simulink model "BDA_DynamicModel_v3"  (R2021b)
settings: Solver=ode23t  StartTime=0.0  StopTime=15  FixedStep=0.000001  MaxStep=1e-5  MinStep=1e-7  RelTol=1e-3
undefined symbols (not defined in the file or in its folder): X, Y, Z
libraries: sm_lib x47, nesl_utility x7
(part 2 of 5)

== matlab function BDA_DynamicModel_v3/Planta/Dinámica Directa/H ==
  data: q2 input; H output; q3 input; q4 input; q5 input; q6 input
function H = H(q2,q3,q4,q5,q6)
%#codegen

%    This function was generated by the Symbolic Math Toolbox version 9.0.
%    28-Nov-2021 14:58:23

t2 = cos(q2);
t3 = cos(q4);
t4 = cos(q5);
t5 = cos(q6);
t6 = sin(q2);
t7 = sin(q4);
t8 = sin(q5);
t9 = sin(q6);
t16 = 9.007199254740992e+15;
t10 = t2.*1.051339e-1;
t11 = t6.*1.051339e-1;
t12 = t4.*5.110348748545983e-1;
t14 = t8.*5.110348748545983e-1;
t15 = t6.*3.235525e-2;
t17 = t2.*3.235525e-2;
t18 = t4.*t7.*8.595599785252598e-1;
t19 = t3.*t9.*8.595599785252598e-1;
t20 = t7.*t8.*8.595599785252598e-1;
t21 = t3.*t5.*8.595599785252598e-1;
t23 = t3.*5.157359871151559e-3;
t24 = t5.*t8.*4.36041e-5;
t25 = t8.*t9.*4.36041e-5;
t26 = (q3.*t16)./9.007199254740992e+15;
t29 = q3.*t16.*1.110223024625157e-16i;
t39 = t5.*1.33637554986e-4;
t40 = t8.*1.33637554986e-4;
t41 = t8.*7.26350557185e-5;
t42 = t9.*7.26350557185e-5;
t43 = t8.*6.1855407534e-5;
t44 = t4.*1.35652563578e-4;
t45 = t3.*t4.*4.990257941055339e-2;
t46 = t5.*t7.*4.990257941055339e-2;
t47 = t7.*t9.*4.990257941055339e-2;
t50 = t4.*t5.*7.26350557185e-5;
t52 = t3.*3.748033925961328e-5;
t53 = t4.*t9.*1.33637554986e-4;
t54 = t3.*t5.*t8.*4.990257941055339e-2;
t55 = t3.*t8.*t9.*4.990257941055339e-2;
t56 = t8.*t9.*4.35810334311e-7;
t61 = t5.*t8.*8.01825329916e-7;
t71 = t6.*5.850606868813307e-5;
t72 = t2.*1.908064240151374e-5;
t74 = t8.*3.161027044821787e-5;
t75 = t8.*3.711904660916042e-5;
t76 = t4.*6.932319085178867e-5;
t77 = t3.*9.395517395143932e-4;
t78 = t7.*9.395517395143932e-4;
t79 = t4.*3.601891949238275e-7;
t80 = t8.*3.601891949238275e-7;
t81 = t3.*5.316843277159623e-5;
t82 = t7.*1.451749445763287e-4;
t83 = t3.*3.746051216014494e-7;
t84 = t3.*1.166015146360021e-4;
t86 = t8.*6.829345118814501e-5;
t89 = t8.*4.203395243364607e-6;
t90 = t7.*5.427853659906482e-4;
t91 = t4.*7.314371377091851e-7;
t92 = t8.*7.314371377091851e-7;
t93 = t3.*t5.*1.148694938939344e-4;
t94 = t5.*3.387428925624357e-6;
t95 = t4.*t7.*6.243418693357491e-5;
t96 = t3.*t9.*6.243418693357491e-5;
t97 = t4.*t7.*1.148694938939344e-4;
t98 = t4.*t7.*5.316843277159623e-5;
t99 = t5.*1.245668607194124e-6;
t100 = t9.*1.745966317740249e-6;
t101 = t9.*1.245668607194124e-6;
t102 = t7.*t8.*1.166015146360021e-4;
t104 = t3.*t4.*5.427853659906482e-4;
t105 = t3.*t8.*5.427853659906482e-4;
t106 = t4.*t7.*6.058377458913066e-7;
t107 = t7.*t8.*6.058377458913066e-7;
t108 = t3.*1.607033050476913e-7;
t109 = t3.*t4.*3.626595104792852e-4;
t110 = t4.*4.0082304082032e-9;
t111 = t5.*t7.*3.626595104792852e-4;
t112 = t7.*t9.*3.626595104792852e-4;
t113 = t4.*t5.*1.745966317740249e-6;
t116 = t3.*6.892169633636063e-7;
t118 = t4.*t9.*3.387428925624357e-6;
t119 = t4.*t9.*(-1.245668607194124e-6);
t120 = t3.*t5.*t8.*3.626595104792852e-4;
t121 = t3.*t8.*t9.*3.626595104792852e-4;
t124 = t8.*5.918087154269792e-7;
t125 = t4.*2.261852897508832e-6;
t132 = t8.*1.87902861198544e-8;
t152 = t4.*3.73789886133219e-7;
t153 = t8.*3.73789886133219e-7;
t154 = t8.*2.148081562157245e-6;
t156 = t7.*6.769412826196288e-6;
t157 = t3.*2.706536467726674e-6;
t158 = t4.*2.048345525044518e-9;
t159 = t3.*2.289498402241797e-6;
t160 = t7.*3.086744386437578e-6;
t162 = t3.*t8.*6.769412826196288e-6;
t163 = t4.*t7.*3.61307032511966e-6;
t165 = t3.*3.445314443599436e-9;
t166 = t4.*t7.*6.287140903818846e-7;
t167 = t7.*t8.*6.287140903818846e-7;
t169 = t3.*t4.*3.086744386437578e-6;
t170 = t3.*t9.*1.500762770582635e-6;
t171 = t3.*t5.*1.070726881249372e-6;
t172 = t3.*t4.*6.668858699921061e-6;
t173 = t3.*t4.*3.624676635982417e-6;
t174 = t3.*t9.*1.070726881249372e-6;
t175 = t5.*t7.*6.668858699921061e-6;
t176 = t7.*6.078899754658124e-9;
t177 = t7.*t9.*3.624676635982417e-6;
t178 = t3.*t5.*2.911698334565516e-6;
t179 = t7.*3.10211731732776e-5;
t180 = t3.*9.392818914088469e-10;
t181 = t7.*9.392818914088469e-10;
t182 = t3.*t4.*3.517249171619401e-8;
t183 = t7.*t8.*3.445314443599436e-9;
t184 = t3.*t8.*3.517249171619401e-8;
t185 = t3.*t5.*t8.*3.624676635982417e-6;
t186 = t3.*t8.*t9.*6.668858699921061e-6;
t190 = t8.*3.024348928260869e-7;
t191 = t4.*1.155885712417937e-6;
t193 = t7.*t8.*1.944198228009988e-6;
t195 = t4.*t7.*5.086950867234759e-7;
t196 = t8.*9.602491515741889e-9;
t207 = t3.*1.615137793366553e-8;
t213 = t4.*t7.*1.615137793366553e-8;
t214 = t3.*2.84449372366336e-5;
t13 = -t11;
t22 = -t20;
t27 = cos(t26);
t28 = sin(t26);
t30 = exp(t29);
t32 = -t29;
t48 = t10+t15;
t49 = -t43;
t57 = -t53;
t58 = -t54;
t59 = t14+t18;
t85 = -t76;
t87 = -t79;
t88 = -t80;
t103 = -t92;
t114 = t4.*t99;
t115 = t4.*t101;
t117 = -t106;
t122 = -t118;
t123 = -t120;
t126 = -t124;
t127 = t23+t45;
t128 = t25+t41;
t129 = t24+t40;
t155 = -t152;
t161 = -t157;
t164 = -t158;
t168 = -t162;
t187 = -t183;
t188 = -t184;
t189 = -t185;
t192 = -t191;
t201 = -t196;
t211 = -t207;
t215 = -t213;
t251 = t39+t42+4.36041e-5;
t266 = t77-8.631097478604537e-5;
t267 = t78+9.554306323645785e-8;
t270 = t82+t108;
t300 = t113+t119;
t314 = t110+t132;
t368 = t56+t61+t89;
t382 = t99+t100+4.35810334311e-7;
t397 = t94+t101+8.01825329916e-7;
t455 = t179+t180+2.208156882018249e-9;
t459 = t181+t214-3.390351827752591e-7;
t31 = t28.^2;
t33 = 1.0./t30;
t34 = t3.*t27;
t35 = t7.*t27;
t36 = t30-1.0;
t51 = t13+t17;
t60 = t12+t22;
t65 = t5.*t59.*(3.0./5.0e+2);
t66 = t9.*t59.*(3.0./5.0e+2);
t67 = t27.*1.273194e-2;
t130 = t5.*t59.*4.36041e-5;
t131 = t9.*t59.*4.36041e-5;
t135 = t27.*3.42298471896e-5;
t136 = t27.*3.07913148585e-5;
t137 = t30.*3.694216783411725e-1;
t138 = t30.*1.305783216588275e-1;
t140 = t27.*3.679077402936e-4;
t194 = t44+t49;
t197 = t3.*t16.*t28.*5.673626844500105e-17;
t198 = t7.*t16.*t28.*5.673626844500105e-17;
t199 = t4.*t16.*t28.*9.543032792050485e-17;
t200 = t8.*t16.*t28.*9.543032792050485e-17;
t203 = t9.*t59.*4.35810334311e-7;
t208 = t50+t57;
t210 = t3.*t16.*t28.*3.404176106700063e-19;
t212 = t5.*t59.*8.01825329916e-7;
t216 = t30.*3.215186923359161e-3;
t218 = t30.*1.345257168956303e-2;
t219 = t27.*8.550795305149304e-7;
t221 = t27.*2.150354518622839e-6;
t228 = t27.*2.380363079699592e-9;
t237 = t16.*t28.*4.87211480085e-18;
t240 = t3.*t16.*t28.*2.479366200131245e-18;
t241 = t7.*t16.*t28.*2.479366200131245e-18;
t242 = t3.*t16.*t28.*7.351481000981246e-18;
t243 = t7.*t16.*t28.*9.810473427588925e-18;
t244 = t7.*t16.*t28.*7.351481000981246e-18;
t245 = t7.*t16.*t28.*4.938358626738924e-18;
t257 = t3.*t16.*t28.*2.47393392290267e-21;
t258 = t30.*1.073174736839591e-5;
t259 = t30.*4.490239736257417e-5;
t262 = t30.*3.887314306731568e-4;
t268 = t16.*t28.*2.127584079327986e-20;
t272 = t16.*t28.*1.611765660673211e-20;
t273 = t8.*t16.*t28.*6.931587185740596e-21;
t274 = t3.*t16.*t28.*7.696420262413979e-21;
t277 = t3.*t16.*t28.*3.509445006623964e-21;
t278 = t4.*t16.*t28.*1.294536862550567e-20;
t279 = t7.*t16.*t28.*5.371403294717661e-20;
t280 = t3.*t16.*t28.*2.472625211857455e-23;
t283 = t8.*t16.*t28.*1.275307569480848e-20;
t284 = t7.*t16.*t28.*9.582443148530891e-21;
t285 = t8.*t16.*t28.*5.902881824626087e-21;
t288 = t4.*t16.*t28.*6.726150146755334e-23;
t289 = t8.*t16.*t28.*6.726150146755334e-23;
t290 = t16.*t28.*1.78416509397307e-23;
t292 = t3.*t16.*t28.*2.503226128461205e-19;
t293 = t7.*t16.*t28.*2.503226128461205e-19;
t294 = t3.*t16.*t28.*1.095358398302466e-19;
t295 = t7.*t16.*t28.*1.06707538424542e-19;
t296 = t7.*t16.*t28.*1.095358398302466e-19;
t298 = t114+t122;
t303 = t3.*t16.*t28.*4.549257716411571e-23;
t304 = t3.*t16.*t28.*1.060741086483328e-23;
t305 = t91+t126;
t306 = t103+t125;
t308 = t16.*t28.*t48.*5.673626844500105e-17;
t311 = t30.*5.594793061269655e-7;
t315 = t30.*2.27206524062708e-6;
t318 = t30.*2.515092356455324e-9;
t322 = t16.*t28.*2.00574854081142e-22;
t323 = t16.*t28.*2.258468230849856e-22;
t324 = t16.*t28.*6.331121467597849e-23;
t326 = t7.*t16.*t28.*1.330815870366286e-21;
t327 = t7.*t16.*t28.*6.699010075846667e-22;
t328 = t4.*t16.*t28.*6.980128590482299e-23;
t329 = t8.*t16.*t28.*6.980128590482299e-23;
t330 = t8.*t16.*t28.*4.011313864537747e-22;
t332 = t7.*t16.*t28.*3.054641854059808e-22;
t333 = t7.*t16.*t28.*6.068308319649908e-22;
t334 = t4.*t16.*t28.*3.825067422357704e-25;
t335 = t3.*t16.*t28.*1.511210377393976e-22;
t340 = t3.*t16.*t28.*4.563917575948183e-22;
t341 = t3.*t16.*t28.*2.274120364292329e-25;
t342 = t16.*t28.*t48.*1.893760189037778e-19;
t343 = t16.*t28.*4.123498135247176e-25;
t346 = t7.*t16.*t28.*3.145845434116526e-21;
t347 = t3.*t16.*t28.*1.279265104253459e-21;
t350 = t7.*t16.*t28.*6.39965864882112e-21;
t351 = t7.*t16.*t28.*7.086968837016952e-25;
t353 = t3.*t16.*t28.*6.199840717099487e-26;
t354 = t7.*t16.*t28.*6.199840717099487e-26;
t360 = t7.*t16.*t28.*1.6195873051144e-24;
t362 = t4.*t16.*t28.*2.158493637172119e-22;
t363 = t8.*t16.*t28.*5.647649977940937e-23;
t367 = t3.*t16.*t28.*1.659646412768137e-22;
t370 = t3.*t16.*t28.*1.066090717454436e-24;
t371 = t16.*t28.*3.909932369564116e-22;
t372 = t8.*t16.*t28.*1.793163166137816e-24;
t373 = t3.*t16.*t28.*2.975797947808626e-21;
t375 = t3.*t16.*t28.*6.22961116251322e-21;
t380 = t16.*t28.*5.699051429514929e-23;
t385 = t16.*t28.*t48.*1.94207379898051e-21;
t387 = t16.*t28.*t48.*1.746984305586406e-21;
t405 = t16.*t28.*1.428206656218648e-22;
t412 = t16.*t28.*t48.*5.091703513734173e-22;
t456 = t81+t87+t104+t107;
t457 = t84+t88+t105+t117;
t458 = t161+t176+2.093791190610393e-6;
t487 = t74+t85+t90+t98+t102;
t580 = t153+t156+t165+t166+t182+t192+t193;
t581 = t155+t160+t167+t188+t190+t195+t211;
t582 = t159+t162+t164+t169+t183+t201+t215;
t37 = t36.^2;
t38 = t35.*(3.0./5.0e+2);
t62 = t5.*t60;
t63 = t9.*t60;
t68 = t34.*2.228474e-2;
t69 = t35.*2.228474e-2;
t70 = t34.*6.562549e-2;
t73 = t35.*4.36041e-5;
t139 = t33.*3.694216783411725e-1;
t141 = t33.*1.305783216588275e-1;
t142 = t34.*1.3117937708872e-3;
t143 = t35.*1.3117937708872e-3;
t144 = t35.*1.35652563578e-4;
t145 = t34.*1.688944904408e-4;
t146 = t35.*6.1855407534e-5;
t147 = t35.*4.35810334311e-7;
t148 = t34.*7.13801892181e-4;
t149 = t35.*1.869599668e-7;
t151 = t35.*8.01825329916e-7;
t205 = -t198;
t206 = -t199;
t217 = t33.*3.215186923359161e-3;
t220 = t33.*1.345257168956303e-2;
t222 = t34.*8.902265954562403e-6;
t223 = t35.*4.427198467956924e-6;
t225 = t35.*2.663570267859459e-6;
t226 = t34.*4.059291428568442e-6;
t227 = t35.*4.0082304082032e-9;
t230 = t34.*4.114486328260564e-5;
t231 = t34.*8.487305697640184e-9;
t232 = t34.*1.092747353151976e-9;
t233 = t35.*1.092747353151976e-9;
t235 = t35.*2.925194867859459e-6;
t236 = t35.*1.87902861198544e-8;
t238 = t35.*3.814770659661843e-5;
t246 = -t241;
t252 = -t243;
t253 = -t244;
t254 = -t245;
t260 = t33.*1.073174736839591e-5;
t261 = t33.*4.490239736257417e-5;
t263 = t33.*3.887314306731568e-4;
t264 = t35.*2.262452815028836e-6;
t265 = t34.*4.33730920504627e-9;
t269 = t35+t197;
t286 = -t278;
t287 = -t279;
t297 = -t284;
t299 = -t293;
t301 = -t295;
t302 = -t296;
t307 = -t304;
t309 = t16.*t28.*t51.*9.543032792050485e-17;
t312 = t33.*5.594793061269655e-7;
t317 = t33.*2.27206524062708e-6;
t319 = t33.*2.515092356455324e-9;
t320 = t46+t55+t65;
t321 = t47+t58+t66;
t325 = -t324;
t331 = -t326;
t336 = -t328;
t338 = -t329;
t344 = -t332;
t345 = -t333;
t348 = -t341;
t349 = -t346;
t352 = t16.*t28.*t51.*3.185302114428987e-19;
t355 = -t350;
t356 = -t351;
t358 = -t353;
t359 = -t354;
t361 = -t360;
t365 = -t362;
t374 = -t373;
t376 = -t375;
t381 = -t380;
t390 = t16.*t28.*t51.*3.266565541972299e-21;
t398 = t16.*t28.*t51.*2.938425274050169e-21;
t413 = t16.*t28.*t51.*8.564238525144865e-22;
t414 = -t412;
t488 = t75+t95+t112+t123+t131;
t489 = t86+t97+t111+t121+t130;
t490 = t16.*t28.*t458.*9.543032792050485e-17;
t594 = t154+t163+t175+t177+t186+t189+t203+t212;
t64 = -t62;
t133 = t21+t63;
t150 = -t149;
t202 = t63.*1.33637554986e-4;
t204 = t62.*7.26350557185e-5;
t224 = -t222;
t229 = -t227;
t234 = -t233;
t239 = -t238;
t247 = t63.*3.387428925624357e-6;
t248 = t62.*1.745966317740249e-6;
t249 = t62.*1.245668607194124e-6;
t250 = t63.*1.245668607194124e-6;
t271 = t34+t205;
t275 = t5.*t269;
t276 = t9.*t269;
t310 = -t309;
t313 = t33.*t37.*7.997968101822611e-3;
t316 = t33.*t37.*5.407940120688672e-3;
t337 = t4.*t269.*4.334075e-2;
t339 = t8.*t269.*4.334075e-2;
t357 = -t352;
t364 = t33.*t37.*2.669585786930656e-5;
t366 = t33.*t37.*1.805078477303827e-5;
t369 = t33.*t37.*1.56270217221073e-4;
t377 = t33.*t37.*t48.*2.196325630278387e-1;
t378 = t33.*t37.*t51.*2.196325630278387e-1;
t383 = t4.*t269.*4.71413003675e-4;
t384 = t8.*t269.*4.71413003675e-4;
t386 = t39.*t269;
t388 = t4.*t269.*3.149723995125e-4;
t389 = t42.*t269;
t396 = -t390;
t401 = -t398;
t404 = t33.*t37.*4.313809179931398e-7;
t406 = t33.*t37.*9.133712910180717e-7;
t407 = t33.*t37.*1.011068305420342e-9;
t408 = t33.*t37.*t48.*7.330961578512107e-4;
t409 = t33.*t37.*t51.*7.330961578512107e-4;
t410 = t33.*t37.*t48.*6.346599179580158e-3;
t415 = t4.*t269.*3.148057791131579e-6;
t416 = t8.*t269.*5.879283844893203e-6;
t417 = t4.*t269.*2.68085975407921e-6;
t418 = t4.*t269.*5.791951861259479e-6;
t419 = t94.*t269;
t420 = t4.*t269.*4.57069415115421e-6;
t422 = t99.*t269;
t423 = t100.*t269;
t424 = t101.*t269;
t426 = t4.*t269.*3.054756263814e-8;
t428 = t8.*t269.*3.054756263814e-8;
t433 = t137+t139+2.61156643317655e-1;
t434 = t138+t141+7.38843356682345e-1;
t438 = t33.*t37.*t48.*7.517989070303108e-6;
t440 = t33.*t37.*t51.*6.762775401369527e-6;
t442 = t33.*t37.*t48.*3.70947298167937e-5;
t443 = t33.*t37.*t48.*4.106249669188362e-8;
t466 = t269.*t314;
t503 = t269.*t459;
t595 = t269.*t582;
t134 = t19+t64;
t209 = -t204;
t255 = -t248;
t256 = -t249;
t281 = t4.*t271;
t282 = t8.*t271;
t291 = -t276;
t379 = -t378;
t393 = t276.*4.35810334311e-7;
t402 = t275.*8.01825329916e-7;
t411 = -t409;
t425 = t91.*t271;
t427 = t92.*t271;
t430 = -t426;
t441 = -t440;
t450 = t48.*t434;
t451 = t51.*t433;
t497 = t237+t308+t310;
t502 = t271.*t455;
t504 = -t503;
t505 = t216+t217+t313+1.819229615328168e-2;
t506 = t218+t220+t316+9.510076620873934e-3;
t528 = t268+t342+t357;
t555 = t323+t385+t396;
t558 = t322+t387+t401;
t563 = t136+t258+t260+t364+6.072279186930818e-5;
t564 = t135+t259+t261+t366+3.174301904745164e-5;
t592 = t219+t311+t312+t404+8.856931883486768e-7;
t596 = -t595;
t639 = t140+t145+t150+t262+t263+t297+t307+t369+2.748073584704864e-4;
t391 = t282.*1.35652563578e-4;
t392 = t281.*1.33637554986e-4;
t394 = t281.*7.26350557185e-5;
t395 = t281.*6.1855407534e-5;
t399 = t281.*7.0482312e-7;
t400 = t282.*7.0482312e-7;
t421 = t281.*4.203395243364607e-6;
t429 = t281.*(-7.314371377091851e-7);
t431 = t282.*4.0082304082032e-9;
t435 = t281.*5.918087154269792e-7;
t436 = t282.*2.261852897508832e-6;
t439 = t281.*1.87902861198544e-8;
t444 = t200+t281;
t445 = t206+t282;
t446 = -t5.*(t199-t282);
t447 = -t9.*(t199-t282);
t452 = -t451;
t460 = t450.*3.33783e-3;
t461 = t451.*3.33783e-3;
t462 = t451.*2.889644e-2;
t465 = t9.*(t199-t282).*(-1.33637554986e-4);
t468 = t5.*(t199-t282).*(-7.26350557185e-5);
t469 = t5.*(t199-t282).*(-4.35810334311e-7);
t470 = t5.*(t199-t282).*7.26350557185e-5;
t471 = t5.*(t199-t282).*4.35810334311e-7;
t473 = t9.*(t199-t282).*(-8.01825329916e-7);
t474 = t451.*3.42298471896e-5;
t475 = t450.*3.07913148585e-5;
t477 = t451.*1.688944904408e-4;
t479 = t451.*1.869599668e-7;
t481 = t9.*(t199-t282).*(-3.387428925624357e-6);
t482 = t5.*(t199-t282).*(-1.745966317740249e-6);
t483 = -t99.*(t199-t282);
t484 = -t101.*(t199-t282);
t485 = t5.*(t199-t282).*1.745966317740249e-6;
t486 = t5.*(t199-t282).*1.245668607194124e-6;
t493 = -t306.*(t199-t282);
t496 = t306.*(t199-t282);
t498 = t3.*t497;
t499 = t7.*t497;
t507 = t3.*t505;
t508 = t7.*t505;
H = ft_1({t105,t106,t109,t116,t127,t128,t129,t133,t134,t142,t143,t144,t146,t147,t148,t151,t158,t159,t16,t168,t169,t170,t171,t172,t173,t174,t178,t187,t196,t199,t2,t202,t208,t209,t210,t213,t221,t222,t223,t224,t225,t226,t227,t228,t229,t230,t231,t232,t234,t235,t236,t237,t239,t240,t242,t246,t247,t250,t251,t252,t253,t254,t255,t256,t257,t264,t265,t266,t267,t268,t269,t27,t270,t271,t272,t273,t274,t275,t276,t277,t28,t280,t282,t283,t285,t286,t287,t288,t289,t290,t291,t292,t294,t298,t299,t3,t300,t301,t302,t303,t305,t306,t31,t314,t315,t317,t318,t319,t320,t321,t325,t326,t327,t329,t330,t331,t334,t335,t336,t337,t338,t339,t340,t341,t343,t344,t345,t347,t348,t349,t355,t356,t358,t359,t361,t362,t363,t365,t367,t368,t370,t371,t372,t374,t376,t377,t379,t38,t381,t382,t383,t384,t386,t388,t389,t39,t391,t392,t393,t394,t395,t397,t399,t4,t40,t400,t402,t405,t406,t407,t408,t41,t410,t411,t413,t414,t415,t416,t417,t418,t419,t42,t420,t421,t422,t423,t424,t425,t426,t427,t428,t429,t43,t430,t431,t435,t436,t438,t439,t44,t441,t442,t443,t444,t446,t447,t45,t450,t452,t455,t456,t458,t459,t460,t461,t462,t465,t466,t470,t471,t473,t474,t475,t477,t479,t48,t481,t484,t485,t486,t487,t488,t489,t490,t496,t497,t498,t499,t5,t502,t504,t505,t506,t507,t508,t51,t52,t528,t555,t558,t563,t564,t580,t581,t582,t59,t592,t594,t596,t6,t60,t62,t63,t639,t67,t68,t69,t7,t70,t71,t72,t73,t8,t80,t83,t84,t9,t93,t96});
end
function H = ft_1(ct)
t105 = ct{1};
t106 = ct{2};
t109 = ct{3};
t116 = ct{4};
t127 = ct{5};
t128 = ct{6};
t129 = ct{7};
t133 = ct{8};
t134 = ct{9};
t142 = ct{10};
t143 = ct{11};
t144 = ct{12};
t146 = ct{13};
t147 = ct{14};
t148 = ct{15};
t151 = ct{16};
t158 = ct{17};
t159 = ct{18};
t16 = ct{19};
t168 = ct{20};
t169 = ct{21};
t170 = ct{22};
t171 = ct{23};
t172 = ct{24};
t173 = ct{25};
t174 = ct{26};
t178 = ct{27};
t187 = ct{28};
t196 = ct{29};
t199 = ct{30};
t2 = ct{31};
t202 = ct{32};
t208 = ct{33};
t209 = ct{34};
t210 = ct{35};
t213 = ct{36};
t221 = ct{37};
t222 = ct{38};
t223 = ct{39};
t224 = ct{40};
t225 = ct{41};
t226 = ct{42};
t227 = ct{43};
t228 = ct{44};
t229 = ct{45};
t230 = ct{46};
t231 = ct{47};
t232 = ct{48};
t234 = ct{49};
t235 = ct{50};
t236 = ct{51};
t237 = ct{52};
t239 = ct{53};
t240 = ct{54};
t242 = ct{55};
t246 = ct{56};
t247 = ct{57};
t250 = ct{58};
t251 = ct{59};
t252 = ct{60};
t253 = ct{61};
t254 = ct{62};
t255 = ct{63};
t256 = ct{64};
t257 = ct{65};
t264 = ct{66};
t265 = ct{67};
t266 = ct{68};
t267 = ct{69};
t268 = ct{70};
t269 = ct{71};
t27 = ct{72};
t270 = ct{73};
t271 = ct{74};
t272 = ct{75};
t273 = ct{76};
t274 = ct{77};
t275 = ct{78};
t276 = ct{79};
t277 = ct{80};
t28 = ct{81};
t280 = ct{82};
t282 = ct{83};
t283 = ct{84};
t285 = ct{85};
t286 = ct{86};
t287 = ct{87};
t288 = ct{88};
t289 = ct{89};
t290 = ct{90};
t291 = ct{91};
t292 = ct{92};
t294 = ct{93};
t298 = ct{94};
t299 = ct{95};
t3 = ct{96};
t300 = ct{97};
t301 = ct{98};
t302 = ct{99};
t303 = ct{100};
t305 = ct{101};
t306 = ct{102};
t31 = ct{103};
t314 = ct{104};
t315 = ct{105};
t317 = ct{106};
t318 = ct{107};
t319 = ct{108};
t320 = ct{109};
t321 = ct{110};
t325 = ct{111};
t326 = ct{112};
t327 = ct{113};
t329 = ct{114};
t330 = ct{115};
t331 = ct{116};
t334 = ct{117};
t335 = ct{118};
t336 = ct{119};
t337 = ct{120};
t338 = ct{121};
t339 = ct{122};
t340 = ct{123};
t341 = ct{124};
t343 = ct{125};
t344 = ct{126};
t345 = ct{127};
t347 = ct{128};
t348 = ct{129};
t349 = ct{130};
t355 = ct{131};
t356 = ct{132};
t358 = ct{133};
t359 = ct{134};
t361 = ct{135};
t362 = ct{136};
t363 = ct{137};
t365 = ct{138};
t367 = ct{139};
t368 = ct{140};
t370 = ct{141};
t371 = ct{142};
t372 = ct{143};
t374 = ct{144};
t376 = ct{145};
t377 = ct{146};
t379 = ct{147};
t38 = ct{148};
t381 = ct{149};
t382 = ct{150};
t383 = ct{151};
t384 = ct{152};
t386 = ct{153};
t388 = ct{154};
t389 = ct{155};
t39 = ct{156};
t391 = ct{157};
t392 = ct{158};
t393 = ct{159};
t394 = ct{160};
t395 = ct{161};
t397 = ct{162};
t399 = ct{163};
t4 = ct{164};
t40 = ct{165};
t400 = ct{166};
t402 = ct{167};
t405 = ct{168};
t406 = ct{169};
t407 = ct{170};
t408 = ct{171};
t41 = ct{172};
t410 = ct{173};
t411 = ct{174};
t413 = ct{175};
t414 = ct{176};
t415 = ct{177};
t416 = ct{178};
t417 = ct{179};
t418 = ct{180};
t419 = ct{181};
t42 = ct{182};
t420 = ct{183};
t421 = ct{184};
t422 = ct{185};
t423 = ct{186};
t424 = ct{187};
t425 = ct{188};
t426 = ct{189};
t427 = ct{190};
t428 = ct{191};
t429 = ct{192};
t43 = ct{193};
t430 = ct{194};
t431 = ct{195};
t435 = ct{196};
t436 = ct{197};
t438 = ct{198};
t439 = ct{199};
t44 = ct{200};
t441 = ct{201};
t442 = ct{202};
t443 = ct{203};
t444 = ct{204};
t446 = ct{205};
t447 = ct{206};
t45 = ct{207};
t450 = ct{208};
t452 = ct{209};
t455 = ct{210};
t456 = ct{211};
t458 = ct{212};
t459 = ct{213};
t460 = ct{214};
t461 = ct{215};
t462 = ct{216};
t465 = ct{217};
t466 = ct{218};
t470 = ct{219};
t471 = ct{220};
t473 = ct{221};
t474 = ct{222};
t475 = ct{223};
t477 = ct{224};
t479 = ct{225};
t48 = ct{226};
t481 = ct{227};
t484 = ct{228};
t485 = ct{229};
t486 = ct{230};
t487 = ct{231};
t488 = ct{232};
t489 = ct{233};
t490 = ct{234};
t496 = ct{235};
t497 = ct{236};
t498 = ct{237};
t499 = ct{238};
t5 = ct{239};
t502 = ct{240};
t504 = ct{241};
t505 = ct{242};
t506 = ct{243};
t507 = ct{244};
t508 = ct{245};
t51 = ct{246};
t52 = ct{247};
t528 = ct{248};
t555 = ct{249};
t558 = ct{250};
t563 = ct{251};
t564 = ct{252};
t580 = ct{253};
t581 = ct{254};
t582 = ct{255};
t59 = ct{256};
t592 = ct{257};
t594 = ct{258};
t596 = ct{259};
t6 = ct{260};
t60 = ct{261};
t62 = ct{262};
t63 = ct{263};
t639 = ct{264};
t67 = ct{265};
t68 = ct{266};
t69 = ct{267};
t7 = ct{268};
t70 = ct{269};
t71 = ct{270};
t72 = ct{271};
t73 = ct{272};
t8 = ct{273};
t80 = ct{274};
t83 = ct{275};
t84 = ct{276};
t9 = ct{277};
t93 = ct{278};
t96 = ct{279};
t525 = t52+t93+t96+t109+t202+t209;
t536 = t67+t506;
t546 = -t300.*(t276+t5.*(t199-t282));
t547 = t300.*(t276+t5.*(t199-t282));
t559 = -t382.*(t276+t5.*(t199-t282));
t561 = t382.*(t276+t5.*(t199-t282));
t562 = t83+t170+t171+t173+t250+t255;
t565 = t116+t172+t174+t178+t247+t256;
t573 = t16.*t28.*t555.*9.543032792050485e-17;
t574 = t16.*t28.*t558.*5.673626844500105e-17;
t593 = t27.*t592;
t599 = t379+t450+t505;
t605 = -t580.*(t199-t282);
t403 = -t400;
t432 = -t431;
t437 = -t436;
t448 = t5.*t444.*(3.0./5.0e+2);
t449 = t9.*t444.*(3.0./5.0e+2);
t453 = t5.*t444.*4.36041e-5;
t454 = t9.*t444.*4.36041e-5;
t463 = -t461;
t464 = -t462;
t467 = t9.*t444.*4.35810334311e-7;
t472 = t5.*t444.*8.01825329916e-7;
t476 = -t474;
t478 = -t477;
t480 = -t479;
t491 = t275+t447;
t492 = t305.*t444;
t494 = t291+t446;
t500 = -t499;
t501 = t368.*t444;
t509 = t498.*2.889644e-2;
t510 = t499.*2.889644e-2;
t512 = t499.*1.08769e-2;
t514 = t507.*2.889644e-2;
t515 = t508.*2.889644e-2;
t516 = t507.*1.08769e-2;
t517 = t498.*1.688944904408e-4;
t518 = t499.*6.1855407534e-5;
t519 = t498.*6.678441185616e-4;
t520 = t499.*6.678441185616e-4;
t521 = t499.*1.35652563578e-4;
t526 = t499.*1.869599668e-7;
t529 = t508.*1.688944904408e-4;
t530 = t507.*6.1855407534e-5;
t531 = t507.*6.678441185616e-4;
t532 = t508.*6.678441185616e-4;
t533 = t507.*1.35652563578e-4;
t535 = t507.*1.869599668e-7;
t537 = t8.*t536;
t538 = t4.*t536;
t548 = t41.*t536;
t549 = t43.*t536;
t550 = t44.*t536;
t551 = t40.*t536;
t566 = t69+t242+t508;
t567 = t68+t253+t507;
t568 = t70+t252+t507;
t600 = t377+t452+t506;
t601 = t3.*t599;
t602 = t7.*t599;
t607 = t444.*t581;
t616 = t377+t452+t536;
t625 = -t562.*(t276+t5.*(t199-t282));
t638 = t444.*t594;
t640 = t411+t460+t563;
t495 = -t492;
t511 = -t510;
t513 = -t512;
t522 = -t518;
t523 = -t519;
t524 = -t520;
t527 = -t526;
t534 = -t532;
t539 = -t537;
t540 = t537.*7.26735e-3;
t541 = t538.*1.08769e-2;
t542 = t537.*1.08769e-2;
t545 = t298.*t491;
t552 = t537.*(-7.26350557185e-5);
t553 = t537.*(-6.1855407534e-5);
t554 = t537.*(-1.33637554986e-4);
t556 = t538.*7.0482312e-7;
t557 = t537.*7.0482312e-7;
t560 = t397.*t491;
t569 = t4.*t566;
t570 = t8.*t566;
t571 = t5.*t568;
t572 = t9.*t568;
t587 = t39.*t568;
t588 = t42.*t568;
t597 = t143+t272+t292+t515;
t598 = t142+t290+t299+t514;
t603 = t601.*2.889644e-2;
t604 = t602.*2.889644e-2;
t606 = t601.*1.08769e-2;
t608 = t602.*1.688944904408e-4;
t609 = t601.*6.1855407534e-5;
t610 = t601.*6.678441185616e-4;
t611 = t602.*6.678441185616e-4;
t612 = t601.*1.35652563578e-4;
t615 = t601.*1.869599668e-7;
t617 = t4.*t616;
t618 = t8.*t616;
t626 = t44.*t616;
t627 = t40.*t616;
t628 = t41.*t616;
t629 = t43.*t616;
t633 = t491.*t565;
t641 = t408+t463+t564;
t653 = t148+t285+t286+t301+t391+t395+t516;
t655 = t69+t240+t498+t602;
t658 = t68+t246+t500+t601;
t659 = t70+t254+t500+t601;
t675 = t410+t464+t639;
t676 = t223+t231+t347+t361+t371+t529+t535;
t679 = t438+t441+t475+t476+t592;
t684 = t221+t230+t234+t315+t317+t343+t355+t358+t406+t531+1.606199544935468e-6;
t543 = -t540;
t544 = -t542;
t575 = t570.*1.08769e-2;
t576 = t569.*7.26735e-3;
t577 = t569.*1.08769e-2;
t578 = t571.*7.26735e-3;
t579 = t572.*7.26735e-3;
t583 = t569.*1.33637554986e-4;
t584 = t569.*7.26350557185e-5;
t585 = t569.*6.1855407534e-5;
t586 = t570.*1.35652563578e-4;
t589 = t569.*7.0482312e-7;
t590 = t570.*7.0482312e-7;
t613 = -t611;
t614 = -t612;
t619 = -t618;
t620 = t617.*1.08769e-2;
t621 = t618.*1.08769e-2;
t622 = t618.*7.26735e-3;
t630 = t618.*(-1.33637554986e-4);
t631 = t618.*(-7.26350557185e-5);
t632 = t618.*(-6.1855407534e-5);
t634 = t618.*7.0482312e-7;
t635 = t617.*7.0482312e-7;
t637 = -t633;
t642 = t339+t538+t570;
t643 = t337+t539+t569;
t656 = t4.*t655;
t657 = t8.*t655;
t660 = t5.*t659;
t661 = t9.*t659;
t673 = t39.*t659;
t674 = t42.*t659;
t677 = t143+t272+t294+t509+t604;
t678 = t142+t290+t302+t511+t603;
t680 = t16.*t28.*t676.*9.543032792050485e-17;
t681 = t27.*t679;
t685 = t228+t232+t239+t318+t319+t325+t359+t376+t407+t534+1.778003609304047e-9;
t686 = t271.*t684;
t691 = t148+t285+t286+t287+t391+t395+t513+t606;
t716 = t221+t230+t234+t315+t317+t343+t349+t358+t406+t442+t478+t524+t610+1.606199544935468e-6;
t720 = t223+t231+t340+t356+t371+t517+t527+t608+t615;
t591 = -t589;
t623 = -t621;
t624 = -t622;
t636 = -t634;
t644 = t5.*t642;
t645 = t9.*t642;
t654 = t38+t210+t643;
t662 = t656.*7.26735e-3;
t663 = t656.*1.08769e-2;
t664 = t657.*1.08769e-2;
t665 = t660.*7.26735e-3;
t666 = t661.*7.26735e-3;
t667 = t656.*7.26350557185e-5;
t668 = t656.*6.1855407534e-5;
t669 = t657.*1.35652563578e-4;
t670 = t656.*1.33637554986e-4;
t671 = t656.*7.0482312e-7;
t672 = t657.*7.0482312e-7;
t682 = t144+t274+t289+t384+t399+t541+t575;
t683 = t146+t277+t288+t383+t403+t544+t577;
t687 = t269.*t685;
t692 = t73+t257+t386+t388+t389+t465+t470+t543+t576;
t695 = t339+t617+t657;
t696 = t337+t619+t656;
t706 = t147+t280+t415+t422+t423+t484+t485+t552+t584;
t707 = t151+t303+t418+t419+t424+t481+t486+t554+t583;
t715 = t226+t236+t336+t345+t363+t370+t427+t428+t435+t530+t556+t590;
t717 = t228+t232+t239+t318+t319+t325+t359+t374+t407+t443+t480+t523+t613+1.778003609304047e-9;
t718 = (t199-t282).*(t224+t227+t326+t338+t341+t362-t425+t426+t437-t533-t557+t589);
t721 = t271.*t716;
t724 = t16.*t28.*t720.*9.543032792050485e-17;
t726 = t225+t334+t335+t372+t416+t417+t432+t439+t550+t553+t585+t586;
t646 = -t645;
t647 = t644.*7.26735e-3;
t648 = t645.*7.26735e-3;
t650 = t645.*1.33637554986e-4;
t651 = t644.*7.26350557185e-5;
t688 = -t687;
t689 = t449+t572+t644;
t697 = t5.*t695;
t698 = t9.*t695;
t708 = t38+t210+t696;
t709 = -t706.*(t276+t5.*(t199-t282));
t710 = t706.*(t276+t5.*(t199-t282));
t711 = t491.*t707;
t712 = t222+t229+t329+t331+t348+t365+t425+t430+t436+t533+t557+t591;
t713 = t144+t274+t289+t384+t399+t620+t664;
t714 = t146+t277+t288+t383+t403+t623+t663;
t719 = t444.*t715;
t722 = t269.*t717;
t725 = t73+t257+t386+t388+t389+t465+t470+t624+t662;
t727 = t147+t280+t415+t422+t423+t484+t485+t631+t667;
t728 = t151+t303+t418+t419+t424+t481+t486+t630+t670;
t729 = t269.*t726;
t739 = t224+t227+t327+t338+t341+t362+t426+t429+t437+t521+t614+t636+t671;
t740 = t226+t236+t336+t344+t363+t370+t427+t428+t435+t522+t609+t635+t672;
t744 = t225+t334+t335+t372+t416+t417+t432+t439+t626+t632+t668+t669;
t649 = -t648;
t652 = -t650;
t690 = t448+t571+t646;
t693 = t273+t394+t454+t579+t647;
t699 = -t698;
t700 = t697.*7.26735e-3;
t701 = t698.*7.26735e-3;
t703 = t698.*1.33637554986e-4;
t704 = t697.*7.26350557185e-5;
t723 = -t722;
t730 = t449+t661+t697;
t732 = -t727.*(t276+t5.*(t199-t282));
t733 = t727.*(t276+t5.*(t199-t282));
t734 = t491.*t728;
t741 = -t739.*(t199-t282);
t742 = t739.*(t199-t282);
t743 = t444.*t740;
t745 = t269.*t744;
t694 = t283+t392+t453+t578+t649;
t702 = -t701;
t705 = -t703;
t731 = t448+t660+t699;
t735 = t273+t394+t454+t666+t700;
t737 = t330+t421+t467+t472+t587+t588+t651+t652;
t736 = t283+t392+t453+t665+t702;
t738 = t444.*t737;
t746 = t330+t421+t467+t472+t673+t674+t704+t705;
t747 = t444.*t746;
et1 = t2.*(-6.595899203175001e-4)+t6.*2.143246017993e-3;
et2 = 4.573233567645e-4;
et3 = t71+t72+t573+t574+t681+t721+t723+t724+t733+t734+t742+t743+t745+t747+t497.*t528+t599.*t640+t600.*t641+t616.*t675+t655.*t677+t658.*t678+t659.*t691+t695.*t713+t696.*t714+t708.*t725+t730.*t735+t731.*t736-t51.*(et1+et2);
et4 = t48.*(t2.*2.143246017993e-3+t6.*6.595899203175001e-4+3.222314966007e-4);
et5 = 2.531318772537663e-4;
et6 = t264+t265+t405+t413+t414+t498.*8.631097478604537e-5;
et7 = t499.*(-9.554306323645785e-8);
et8 = t601.*9.554306323645785e-8;
et9 = t602.*8.631097478604537e-5-t3.*t677.*1.264860527128474e-2;
et10 = t7.*t678.*1.264860527128474e-2+t7.*t691.*4.990257941055339e-2+t3.*t717.*8.595599785252598e-1;
et11 = t7.*t716.*8.595599785252598e-1-t3.*t744.*8.595599785252598e-1+t59.*t740+t60.*t739+t59.*t746-t127.*t725-t133.*t728-t134.*t727+t320.*t736+t321.*t735;
et12 = t3.*t16.*t28.*2.332321047271381e-22;
et13 = t7.*t16.*t28.*(-3.621688232723396e-25);
et14 = t3.*t4.*t714.*(-4.990257941055339e-2)-t3.*t8.*t713.*4.990257941055339e-2;
et15 = t31.*2.671802235009627e-6+t71+t72+t593+t680+t686+t688+t710+t711+t718+t719+t729+t738+t268.*t497+t563.*t599+t564.*t600+t597.*t655+t616.*t639+t598.*t658+t653.*t659;
et16 = t682.*t695+t683.*t696+t692.*t708+t693.*t730+t694.*t731+1.896268252195649e-5;
et17 = t31.*1.108156578290307e-5+t593+t680+t686+t688+t710+t711+t718+t719+t729+t738+t505.*t563+t506.*t564+t566.*t597+t567.*t598+t536.*t639+t568.*t653+t642.*t682+t643.*t683;
et18 = t654.*t692+t689.*t693+t690.*t694+1.896268252195649e-5;
et19 = t264+t265+t405+t507.*9.554306323645785e-8;
et20 = t508.*8.631097478604537e-5-t3.*t597.*1.264860527128474e-2;
et21 = t7.*t598.*1.264860527128474e-2+t7.*t653.*4.990257941055339e-2+t3.*t685.*8.595599785252598e-1;
et22 = t7.*t684.*8.595599785252598e-1-t3.*t726.*8.595599785252598e-1+t59.*t715+t59.*t737-t127.*t692-t133.*t707-t134.*t706+t320.*t694+t321.*t693+t60.*(t224+t227+t326+t338+t341+t362-t425+t426+t437-t533-t557+t589);
et23 = t3.*t16.*t28.*6.53749082458021e-22;
et24 = t7.*t16.*t28.*(-8.276655957852335e-25);
et25 = t3.*t4.*t683.*(-4.990257941055339e-2)-t3.*t8.*t682.*4.990257941055339e-2;
et26 = t3.*(-1.383134525074107e-6);
et27 = t7.*3.106529775375363e-9;
et28 = t3.*t266.*1.264860527128474e-2+t7.*t267.*1.264860527128474e-2+t3.*t459.*8.595599785252598e-1;
et29 = t7.*t455.*8.595599785252598e-1+t7.*t487.*4.990257941055339e-2+t45.*t456+t3.*t582.*8.595599785252598e-1+t59.*t581-t60.*t580+t127.*t525+t59.*t594+t134.*t562+t133.*t565+t320.*t489+t321.*t488;
et30 = t3.*t8.*(t80-t84-t105+t106).*(-4.990257941055339e-2);
et31 = 1.284998062810757e-6;
et32 = t3.*(-2.514380437799477e-6);
et33 = t62.*4.35810334311e-7-t63.*8.01825329916e-7+t158+t168+t187+t196+t213;
et34 = t3.*t4.*(-5.262701449313289e-6);
et35 = t3.*t5.*(-6.892169633636063e-7);
et36 = t3.*t9.*(-3.746051216014494e-7)-t5.*t565-t9.*t562;
et37 = t458-t3.*t314.*8.595599785252598e-1-t127.*t208-t59.*t305+t60.*t306+t59.*t368-t133.*t298-t134.*t300+t128.*t321+t129.*t320+t7.*(t43-t44).*4.990257941055339e-2;
et38 = t3.*t4.^2.*(-3.517249171619401e-8);
et39 = t3.*t8.^2.*(-3.517249171619401e-8);
et40 = t5.*8.01825329916e-7+t9.*4.35810334311e-7+t9.*t382+t5.*t397;
et41 = 2.925194867859459e-6;
mt1 = [et3+et4+et5,et15+et16,t381+t413+t414+t490+t502+t504+t596+t605+t607+t625+t637+t638+t270.*t616-t266.*t655+t267.*t658+t487.*t659-t456.*t696+t488.*t730+t489.*t731-t525.*t708+t695.*(t80-t84-t105+t106)];
mt2 = [t466+t495+t496+t501+t545+t547+t720+t4.*t696.*7.0482312e-7+t8.*t695.*7.0482312e-7+t128.*t730+t129.*t731+t208.*t708+t659.*(t43-t44),t560+t561+t744+t251.*t708,t746];
mt3 = [t71+t72+t573+t574+t681+t721+t723+t724+t733+t734+t742+t743+t745+t747+t237.*t528+t505.*t640+t506.*t641+t536.*t675+t566.*t677+t567.*t678+t568.*t691+t642.*t713+t643.*t714+t654.*t725+t689.*t735+t690.*t736+1.896268252195649e-5,et17+et18];
mt4 = [t381+t490+t502+t504+t596+t605+t607+t625+t637+t638+t270.*t536-t266.*t566+t267.*t567+t487.*t568-t456.*t643+t488.*t689+t489.*t690-t525.*t654+t642.*(t80-t84-t105+t106)];
mt5 = [t466+t495+t496+t501+t545+t547+t676+t4.*t643.*7.0482312e-7+t8.*t642.*7.0482312e-7+t128.*t689+t129.*t690+t208.*t654+t568.*(t43-t44),t560+t561+t726+t251.*t654,t737,et6+et7+et8+et9+et10+et11+et12+et13+et14,et19+et20+et21+et22+et23+et24+et25];
mt6 = [et26+et27+et28+et29+et30+et31,et37+et38+et39,t158-t159+t168-t169+t187+t196+t213-t127.*t251-t134.*t382-t133.*t397,t594,t720+t4.*t739+t8.*t740+t8.*t746+t4.*t5.*t727-t4.*t9.*t728+t5.*t8.*t736.*(3.0./5.0e+2)+t8.*t9.*t735.*(3.0./5.0e+2),t676+t8.*t715+t8.*t737+t4.*(t224+t227+t326+t338+t341+t362-t425+t426+t437-t533-t557+t589)+t5.*t8.*t694.*(3.0./5.0e+2)+t8.*t9.*t693.*(3.0./5.0e+2)+t4.*t5.*t706-t4.*t9.*t707,t458-t4.*t580+t8.*t581+t8.*t594+t5.*t8.*t489.*(3.0./5.0e+2)+t8.*t9.*t488.*(3.0./5.0e+2)-t4.*t5.*t562+t4.*t9.*t565];
mt7 = [t4.*t306-t8.*t305+t8.*t368+t5.*t8.*t129.*(3.0./5.0e+2)+t8.*t9.*t128.*(3.0./5.0e+2)+t4.*t5.*t300-t4.*t9.*t298+4.097159105249182e-6,t314+t4.*t5.*t382-t4.*t9.*t397,t368];
mt8 = [t235+t334+t367+t372+t393+t402+t416+t420+t432+t439+t471+t473-t618.*1.05459507534e-4+t626+t656.*1.05459507534e-4+t669+t5.*t728+t9.*t727];
mt9 = [t235+t334+t367+t372+t393+t402+t416+t420+t432+t439+t471+t473-t537.*1.05459507534e-4+t550+t569.*1.05459507534e-4+t586+t5.*t707+t9.*t706,et32+et33+et34+et35+et36];
mt10 = [t314+t4.*t5.*4.35810334311e-7-t4.*t9.*8.01825329916e-7+t5.*t298+t9.*t300,et40+et41,0.0,t746,t737,t594,t368,0.0];
mt11 = [4.203395243364607e-6];
H = real(reshape([mt1,mt2,mt3,mt4,mt5,mt6,mt7,mt8,mt9,mt10,mt11],6,6));
end
